simulink model "ICs_non_Zero_2ODE_EX4"  (Simulink 8.0)
settings: Solver=ode45  StartTime=pi/2  StopTime=2*pi  RelTol=1e-3
settings Model: Creator=David  LastModifiedBy=David
settings DataIOCC: SignalLoggingSaveFormat=ModelDataLogs
settings DebuggingCC: FcnCallInpInsideContextMsg=UseLocalSettings
settings GRTTargetCC: CombineOutputUpdateFcns=off  GRTInterface=on

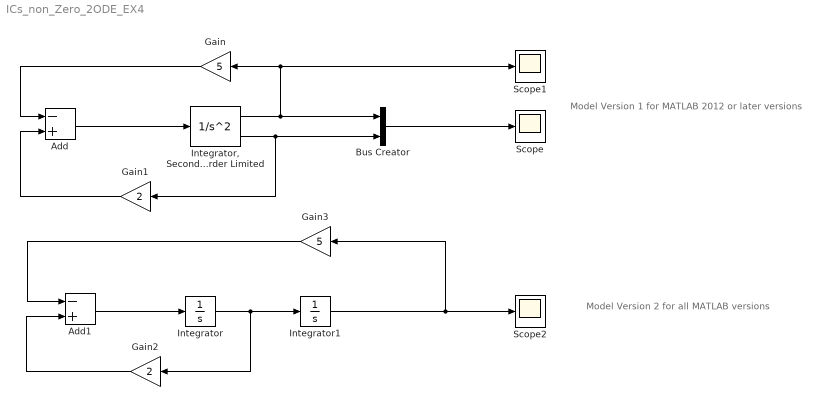
== system ICs_non_Zero_2ODE_EX4 ==
  note: Model Version 2 for all MATLAB versions
  note: Model Version 1 for MATLAB 2012 or later versions
  Add : Sum  Inputs=-+
  Add1 : Sum  Inputs=-+
  Bus Creator : BusCreator  Inputs=2
  Gain : Gain  Gain=5
  Gain1 : Gain  Gain=2
  Gain2 : Gain  Gain=2
  Gain3 : Gain  Gain=5
  Integrator : Integrator  InitialCondition=2
  "Integrator, Second-Order Limited" : SecondOrderIntegrator  UpperLimitX=1  LowerLimitX=0  ICDXDT=2
  Integrator1 : Integrator
  Scope : Scope
  Scope1 : Scope
  Scope2 : Scope
      settings: SaveName=ScopeData2
  wires:
  Add/1 -> "Integrator, Second-Order Limited"/1
  "Integrator, Second-Order Limited"/1 -> Bus Creator/1, Scope1/1, Gain/1
  Gain/1 -> Add/1
  "Integrator, Second-Order Limited"/2 -> Gain1/1, Bus Creator/2
  Gain1/1 -> Add/2
  Bus Creator/1 -> Scope/1
  Add1/1 -> Integrator/1
  Integrator/1 -> Integrator1/1, Gain2/1
  Gain2/1 -> Add1/2
  Integrator1/1 -> Scope2/1, Gain3/1
  Gain3/1 -> Add1/1
